simulink model "velModel1"  (R2021b)
settings: Solver=ode5  StartTime=0.0  StopTime=runT  FixedStep=dt5k  RelTol=1e-3
InitFcn:
  | velInit1;
values from neighbouring files (symbols this model uses):
  Bm = bm * gearRatio * gearRatio    (= 2.601)    [velInit1.m]
  den1cCL = cell2mat(velModelConTFCL.Denominator)    [velInit1.m]
  den1d = cell2mat(velModelDisTF.Denominator)    [velInit1.m]
  den2d = cell2mat(velModelDisTFCL.Denominator)    [velInit1.m]
  denEd = cell2mat(sysEdisTF.Denominator)    [velInit1.m]
  dt1k = 0.001    [velInit1.m]
  dt5k = 1/5000    (= 0.0002)    [velInit1.m]
  Jm = jm * gearRatio * gearRatio    (= 0.023968215)    [velInit1.m]
  kp = 50    [velInit1.m]
  num1cCL = cell2mat(velModelConTFCL.Numerator)    [velInit1.m]
  num1d = cell2mat(velModelDisTF.Numerator)    [velInit1.m]
  num2d = cell2mat(velModelDisTFCL.Numerator)    [velInit1.m]
  numEd = cell2mat(sysEdisTF.Numerator)    [velInit1.m]
  q0 = 0    [velInit1.m]
  seedIndex = floor(rand * 10000)    [velInit1.m]
undefined symbols (not defined in the file or in its folder): DiscIntNeverNeededParam
settings Model: Creator=86135  LastModifiedBy=86135
settings DebuggingCC: AlgebraicLoopMsg=none

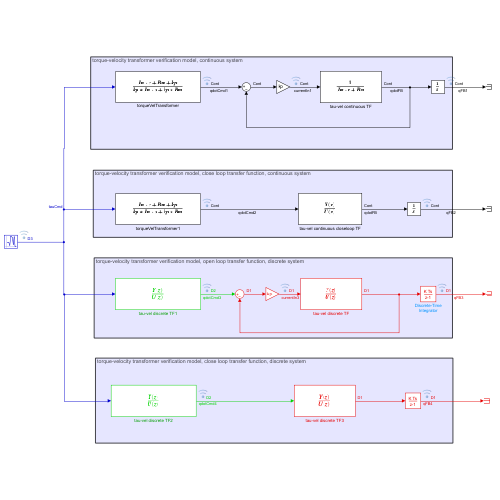
[thumbnail: Simulink's stored preview of the top-level diagram]
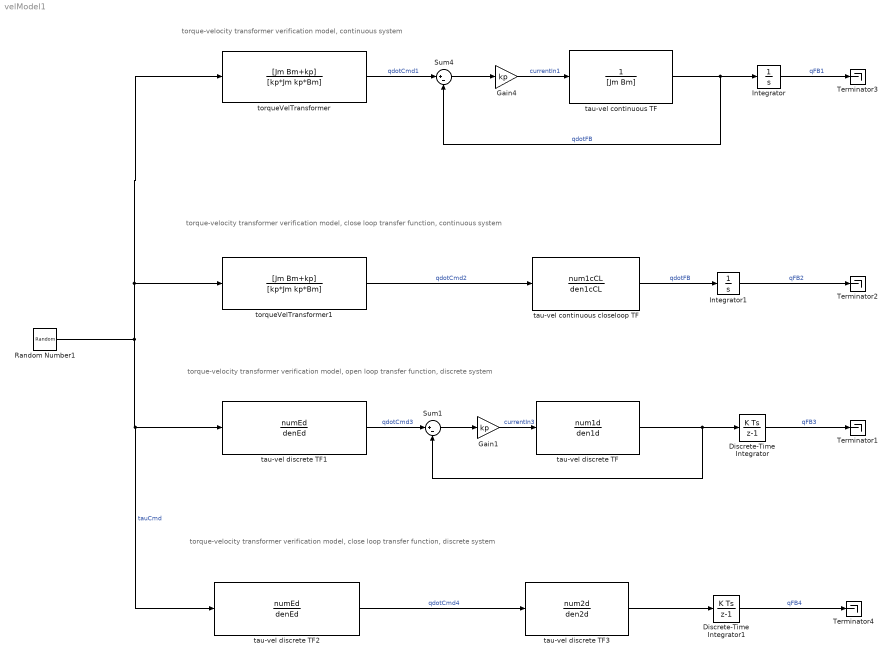
== system velModel1 ==
  note: torque-velocity transformer verification model, close loop transfer function, discrete system
  note: torque-velocity transformer verification model, open loop transfer function, discrete system
  note: torque-velocity transformer verification model, close loop transfer function, continuous system
  note: torque-velocity transformer verification model, continuous system
  Discrete-Time Integrator : DiscreteIntegrator  InitialCondition=q0  SampleTime=dt5k  ICPrevOutput=DiscIntNeverNeededParam  ICPrevScaledInput=DiscIntNeverNeededParam
  Discrete-Time Integrator1 : DiscreteIntegrator  InitialCondition=q0  SampleTime=dt5k  ICPrevOutput=DiscIntNeverNeededParam  ICPrevScaledInput=DiscIntNeverNeededParam
  Gain1 : Gain  Gain=kp
  Gain4 : Gain  Gain=kp
  Integrator : Integrator
  Integrator1 : Integrator  InitialCondition=q0
  Random Number1 : RandomNumber  Variance=10  Seed=seedIndex  SampleTime=0.2
  Sum1 : Sum  Inputs=|+-
  Sum4 : Sum  Inputs=|+-
  Terminator{1..4} (4 alike) : Terminator
  tau-vel continuous TF : TransferFcn  Denominator=[Jm Bm]
  tau-vel continuous closeloop TF : TransferFcn  Numerator=num1cCL  Denominator=den1cCL
  tau-vel discrete TF : DiscreteTransferFcn  Numerator=num1d  Denominator=den1d  SampleTime=dt5k
  tau-vel discrete TF1 : DiscreteTransferFcn  Numerator=numEd  Denominator=denEd  SampleTime=dt1k
  tau-vel discrete TF2 : DiscreteTransferFcn  Numerator=numEd  Denominator=denEd  SampleTime=dt1k
  tau-vel discrete TF3 : DiscreteTransferFcn  Numerator=num2d  Denominator=den2d  SampleTime=dt5k
  torqueVelTransformer : TransferFcn  Numerator=[Jm Bm+kp]  Denominator=[kp*Jm kp*Bm]
  torqueVelTransformer1 : TransferFcn  Numerator=[Jm Bm+kp]  Denominator=[kp*Jm kp*Bm]
  wires:
  Random Number1/1 -> torqueVelTransformer/1, torqueVelTransformer1/1, tau-vel discrete TF2/1, tau-vel discrete TF1/1  "tauCmd"
  torqueVelTransformer/1 -> Sum4/1  "qdotCmd1"
  Sum4/1 -> Gain4/1
  tau-vel continuous TF/1 -> Integrator/1, Sum4/2  "qdotFB"
  Gain4/1 -> tau-vel continuous TF/1  "currentIn1"
  Integrator/1 -> Terminator3/1  "qFB1"
  Discrete-Time Integrator/1 -> Terminator1/1  "qFB3"
  torqueVelTransformer1/1 -> tau-vel continuous closeloop TF/1  "qdotCmd2"
  tau-vel continuous closeloop TF/1 -> Integrator1/1  "qdotFB"
  Integrator1/1 -> Terminator2/1  "qFB2"
  tau-vel discrete TF1/1 -> Sum1/1  "qdotCmd3"
  Gain1/1 -> tau-vel discrete TF/1  "currentIn3"
  tau-vel discrete TF2/1 -> tau-vel discrete TF3/1  "qdotCmd4"
  tau-vel discrete TF3/1 -> Discrete-Time Integrator1/1
  Discrete-Time Integrator1/1 -> Terminator4/1  "qFB4"
  Sum1/1 -> Gain1/1
  tau-vel discrete TF/1 -> Discrete-Time Integrator/1, Sum1/2
